simulink model "WSCC_9bus_distributed"  (R2018a)
settings: Solver=ode3  StartTime=0.0  StopTime=1  FixedStep=Ts  MaxStep=1e-4  RelTol=1e-3
InitFcn:
  | Ts=50e-6;
  | Freq=60;
undefined symbols (not defined in the file or in its folder): gcbh, i, phase, sps_rtmsupport
libraries: powerlib x105, spsVIMeasurementModel x81, library x28, sps_avr x9, CoSiF x7
(part 3 of 5)

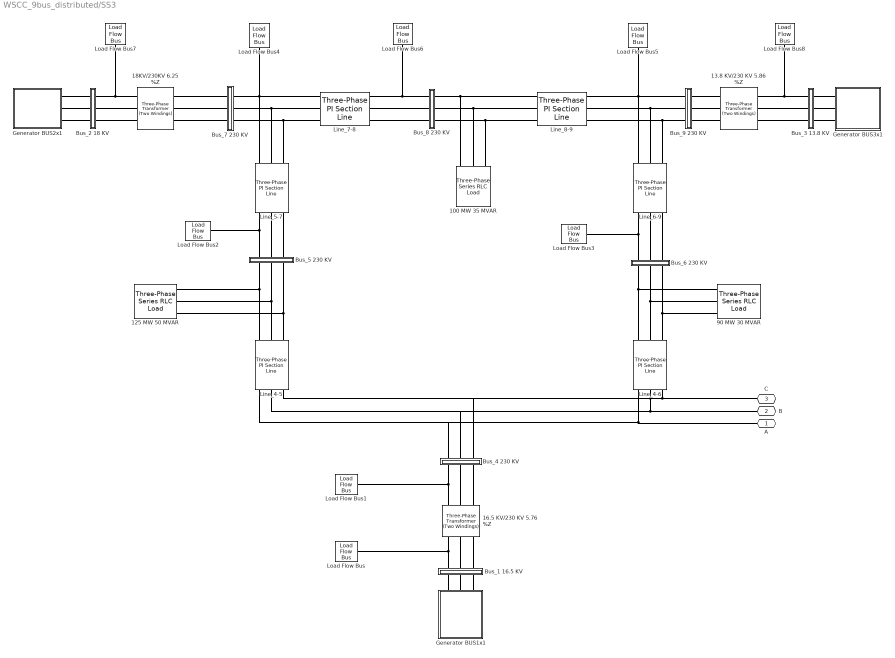
== system WSCC_9bus_distributed/SS3 ==
  100 MW 35 MVAR : powerlib/Elements/Three-Phase Series RLC Load  LConnTagsString=A|B|C  Configuration=Y (grounded)  NominalVoltage=(230000)*1.01601  Vabc=[1e3 1e3 1e3]  Vabcp=[1e3 1e3 1e3]  NominalFrequency=60  UnbalancedPower=off  ActivePower=100e6  InductivePower=35e6  CapacitivePower=0  Pabc=[10e3 9e3 11e3]  QLabc=[100 90 110]  QCabc=[100 90 110]  Pabcp=[10e3 9e3 11e3]  QLabcp=[100 90 110]  QCabcp=[100 90 110]  Measurements=Branch voltages and currents  LoadType=constant PQ
  125 MW 50 MVAR : powerlib/Elements/Three-Phase Series RLC Load  LConnTagsString=A|B|C  Configuration=Y (grounded)  NominalVoltage=(230000)*0.996126  Vabc=[1e3 1e3 1e3]  Vabcp=[1e3 1e3 1e3]  NominalFrequency=60  UnbalancedPower=off  ActivePower=125e6  InductivePower=50e6  CapacitivePower=0  Pabc=[10e3 9e3 11e3]  QLabc=[100 90 110]  QCabc=[100 90 110]  Pabcp=[10e3 9e3 11e3]  QLabcp=[100 90 110]  QCabcp=[100 90 110]  Measurements=Branch voltages and currents  LoadType=constant PQ
  13.8 KV/230 KV 5.86 %Z : powerlib/Elements/Three-Phase Transformer (Two Windings)  Winding1Connection=Yg  Winding2Connection=Yg  CoreType=Three single-phase transformers  SetSaturation=off  Hysteresis=off  DataFile='hysteresis'  SetInitialFlux=off  Measurements=None  UNITS=pu  NominalPower=[ 128e6 , 60 ]  Winding1=[ 13.8e3 , 1e-6 , 0.0 ]  Winding2=[ 230e3 , 1e-6, 0.075008 ]  Rm=inf  Lm=inf  L0=0.5  Saturation=[ 0,0 ; 0.0024,1.2 ; 1.0,1.52 ]  InitialFluxes=[ 0.8 , -0.8 , 0.7 ]  MoreParameters=off  BreakLoop=off  DataType=off  TransfoNumber=1
  "16.5 KV/230 KV 5.76 %Z     " : powerlib/Elements/Three-Phase Transformer (Two Windings)  Winding1Connection=Yg  Winding2Connection=Yg  CoreType=Three single-phase transformers  SetSaturation=off  Hysteresis=off  DataFile='hysteresis'  SetInitialFlux=off  Measurements=None  UNITS=pu  NominalPower=[ 247.5e6 , 60 ]  Winding1=[ 16.5e3 , 1e-6, 0.0 ]  Winding2=[ 230e3 ,1e-6, 0.14256 ]  Rm=inf  Lm=inf  L0=0.5  Saturation=[ 0,0 ; 0.0024,1.2 ; 1.0,1.52 ]  InitialFluxes=[ 0.8 , -0.8 , 0.7 ]  MoreParameters=off  BreakLoop=off  DataType=off  TransfoNumber=1
  18KV/230KV 6.25 %Z : powerlib/Elements/Three-Phase Transformer (Two Windings)  Winding1Connection=Yg  Winding2Connection=Yg  CoreType=Three single-phase transformers  SetSaturation=off  Hysteresis=off  DataFile='hysteresis'  SetInitialFlux=off  Measurements=None  UNITS=pu  NominalPower=[ 192e6 , 60 ]  Winding1=[ 18e3 , 1e-6 , 0.0 ]  Winding2=[ 230e3 , 1e-6, 0.12 ]  Rm=inf  Lm=inf  L0=0.5  Saturation=[ 0,0 ; 0.0024,1.2 ; 1.0,1.52 ]  InitialFluxes=[ 0.8 , -0.8 , 0.7 ]  MoreParameters=off  BreakLoop=off  DataType=off  TransfoNumber=1
  90 MW 30 MVAR : powerlib/Elements/Three-Phase Series RLC Load  LConnTagsString=A|B|C  Configuration=Y (grounded)  NominalVoltage=(230000)*1.01311  Vabc=[1e3 1e3 1e3]  Vabcp=[1e3 1e3 1e3]  NominalFrequency=60  UnbalancedPower=off  ActivePower=90e6  InductivePower=30e6  CapacitivePower=0  Pabc=[10e3 9e3 11e3]  QLabc=[100 90 110]  QCabc=[100 90 110]  Pabcp=[10e3 9e3 11e3]  QLabcp=[100 90 110]  QCabcp=[100 90 110]  Measurements=Branch voltages and currents  LoadType=constant PQ
  Bus_1 16.5 KV : Subsystem  DialogController=POWERSYS.PowerSysDialog  LoadFcn=sps_rtmsupport('LoadFcn',gcbh);  StartFcn=sps_rtmsupport('StartFcn',gcbh);  StopFcn=sps_rtmsupport('StopFcn',gcbh);  mask(Three-Phase VI Measurement){VoltageMeasurement=phase-to-phase, SetLabelV=on, LabelV=ss3_Vabc_1, Vpu=off, VpuLL=off, CurrentMeasurement=yes, SetLabelI=on, LabelI=ss3_Iabc_1, Ipu=off, Pbase=100e6, Vbase=16.5e3, OutputType=Complex, PhasorSimulation=off, PSBequivalent=0}
      mask prompts: VoltageMeasurement "Voltage measurement"; SetLabelV "Use a label"; LabelV "Signal label  (use a From block to collect this signal)"; Vpu "Voltages in pu,  based on peak value of nominal phase-to-ground voltage"; VpuLL "Voltages in pu,  based on peak value of nominal phase-to-phase  voltage"; CurrentMeasurement "Current measurement"; SetLabelI "Use a label"; LabelI "Signal label  (use a From block to collect this signal)"; Ipu "Currents in pu"; Pbase "Base power ( VA 3 phase)"; Vbase "Nominal voltage used for pu measurement (Vrms phase-phase) :"; OutputType "Output signals in:"; PhasorSimulation "Phasor simulation (internal use)"; PSBequivalent "Equivalent circuit (internal use)"
      mask help:
      | Ideal three-phase voltage and current measurements.
      |
      | The block can output the voltages and currents in per unit values or in volts and amperes.
      mask init: same as WSCC_9bus_distributed/SS1/Bus_1 16.5 KV
      settings: CopyFcn=sps_rtmsupport('CopyFcn',gcbh); powericon('ThreePhaseVIMeasurementCopy',gcb)  DeleteFcn=sps_rtmsupport('DeleteFcn',gcbh);  UndoDeleteFcn=sps_rtmsupport('UndoDeleteFcn',gcbh);  ModelCloseFcn=sps_rtmsupport('ModelCloseFcn',gcbh);  PreSaveFcn="sps_rtmsupport('PreSaveFcn',gcbh);  set_param(gcb,'LinkStatus','restore')"  PostSaveFcn=sps_rtmsupport('PostSaveFcn',gcbh);  NameChangeFcn=sps_rtmsupport('NameChangeFcn',gcbh);  PreCopyFcn=sps_rtmsupport('PreCopyFcn',gcbh);  OpenFcn=sps_rtmsupport('OpenFcn',gcbh, [1 2 4 5 6 7 9 -12 13]);  CloseFcn=sps_rtmsupport('CloseFcn',gcbh);  PreDeleteFcn=sps_rtmsupport('PreDeleteFcn',gcbh);
      mask Help: helpview(psbhelp)
      mask TypeOptions VoltageMeasurement: no | phase-to-ground | phase-to-phase
      mask Callback VoltageMeasurement: powericon('ThreePhaseVIMeasurementCback',gcb,'Vselector');
      mask Callback SetLabelV: powericon('ThreePhaseVIMeasurementCback',gcb,'');
      mask Callback Vpu: powericon('ThreePhaseVIMeasurementCback',gcb,'Vpu');
      mask Callback VpuLL: powericon('ThreePhaseVIMeasurementCback',gcb,'VpuLL');
      mask TypeOptions CurrentMeasurement: no | yes
      mask Callback CurrentMeasurement: powericon('ThreePhaseVIMeasurementCback',gcb,'');
      mask Callback SetLabelI: powericon('ThreePhaseVIMeasurementCback',gcb,'');
      mask Callback LabelI: powericon('ThreePhaseVIMeasurementCback',gcb,'');
      mask Callback Ipu: powericon('ThreePhaseVIMeasurementCback',gcb,'');
      mask TypeOptions OutputType: Complex | Real-Imag | Magnitude-Angle | Magnitude
  Bus_2 18 KV : Subsystem  DialogController=POWERSYS.PowerSysDialog  LoadFcn=sps_rtmsupport('LoadFcn',gcbh);  StartFcn=sps_rtmsupport('StartFcn',gcbh);  StopFcn=sps_rtmsupport('StopFcn',gcbh);  mask(Three-Phase VI Measurement){VoltageMeasurement=phase-to-phase, SetLabelV=on, LabelV=ss3_Vabc_2, Vpu=off, VpuLL=off, CurrentMeasurement=yes, SetLabelI=on, LabelI=ss3_Iabc_2, Ipu=off, Pbase=100e6, Vbase=18e3, OutputType=Complex, PhasorSimulation=off, PSBequivalent=0}
      mask prompts: VoltageMeasurement "Voltage measurement"; SetLabelV "Use a label"; LabelV "Signal label  (use a From block to collect this signal)"; Vpu "Voltages in pu,  based on peak value of nominal phase-to-ground voltage"; VpuLL "Voltages in pu,  based on peak value of nominal phase-to-phase  voltage"; CurrentMeasurement "Current measurement"; SetLabelI "Use a label"; LabelI "Signal label  (use a From block to collect this signal)"; Ipu "Currents in pu"; Pbase "Base power ( VA 3 phase)"; Vbase "Nominal voltage used for pu measurement (Vrms phase-phase) :"; OutputType "Output signals in:"; PhasorSimulation "Phasor simulation (internal use)"; PSBequivalent "Equivalent circuit (internal use)"
      mask help:
      | Ideal three-phase voltage and current measurements.
      |
      | The block can output the voltages and currents in per unit values or in volts and amperes.
      mask init: same as WSCC_9bus_distributed/SS1/Bus_1 16.5 KV
      settings: CopyFcn=sps_rtmsupport('CopyFcn',gcbh); powericon('ThreePhaseVIMeasurementCopy',gcb)  DeleteFcn=sps_rtmsupport('DeleteFcn',gcbh);  UndoDeleteFcn=sps_rtmsupport('UndoDeleteFcn',gcbh);  ModelCloseFcn=sps_rtmsupport('ModelCloseFcn',gcbh);  PreSaveFcn="sps_rtmsupport('PreSaveFcn',gcbh);  set_param(gcb,'LinkStatus','restore')"  PostSaveFcn=sps_rtmsupport('PostSaveFcn',gcbh);  NameChangeFcn=sps_rtmsupport('NameChangeFcn',gcbh);  PreCopyFcn=sps_rtmsupport('PreCopyFcn',gcbh);  OpenFcn=sps_rtmsupport('OpenFcn',gcbh, [1 2 4 5 6 7 9 -12 13]);  CloseFcn=sps_rtmsupport('CloseFcn',gcbh);  PreDeleteFcn=sps_rtmsupport('PreDeleteFcn',gcbh);
      mask Help: helpview(psbhelp)
      mask TypeOptions VoltageMeasurement: no | phase-to-ground | phase-to-phase
      mask Callback VoltageMeasurement: powericon('ThreePhaseVIMeasurementCback',gcb,'Vselector');
      mask Callback SetLabelV: powericon('ThreePhaseVIMeasurementCback',gcb,'');
      mask Callback Vpu: powericon('ThreePhaseVIMeasurementCback',gcb,'Vpu');
      mask Callback VpuLL: powericon('ThreePhaseVIMeasurementCback',gcb,'VpuLL');
      mask TypeOptions CurrentMeasurement: no | yes
      mask Callback CurrentMeasurement: powericon('ThreePhaseVIMeasurementCback',gcb,'');
      mask Callback SetLabelI: powericon('ThreePhaseVIMeasurementCback',gcb,'');
      mask Callback LabelI: powericon('ThreePhaseVIMeasurementCback',gcb,'');
      mask Callback Ipu: powericon('ThreePhaseVIMeasurementCback',gcb,'');
      mask TypeOptions OutputType: Complex | Real-Imag | Magnitude-Angle | Magnitude
  Bus_3 13.8 KV : Subsystem  DialogController=POWERSYS.PowerSysDialog  LoadFcn=sps_rtmsupport('LoadFcn',gcbh);  StartFcn=sps_rtmsupport('StartFcn',gcbh);  StopFcn=sps_rtmsupport('StopFcn',gcbh);  mask(Three-Phase VI Measurement){VoltageMeasurement=phase-to-phase, SetLabelV=on, LabelV=ss3_Vabc_3, Vpu=off, VpuLL=off, CurrentMeasurement=yes, SetLabelI=on, LabelI=ss3_Iabc_3, Ipu=off, Pbase=100e6, Vbase=13.8e3, OutputType=Complex, PhasorSimulation=off, PSBequivalent=0}
      mask prompts: VoltageMeasurement "Voltage measurement"; SetLabelV "Use a label"; LabelV "Signal label  (use a From block to collect this signal)"; Vpu "Voltages in pu,  based on peak value of nominal phase-to-ground voltage"; VpuLL "Voltages in pu,  based on peak value of nominal phase-to-phase  voltage"; CurrentMeasurement "Current measurement"; SetLabelI "Use a label"; LabelI "Signal label  (use a From block to collect this signal)"; Ipu "Currents in pu"; Pbase "Base power ( VA 3 phase)"; Vbase "Nominal voltage used for pu measurement (Vrms phase-phase) :"; OutputType "Output signals in:"; PhasorSimulation "Phasor simulation (internal use)"; PSBequivalent "Equivalent circuit (internal use)"
      mask help:
      | Ideal three-phase voltage and current measurements.
      |
      | The block can output the voltages and currents in per unit values or in volts and amperes.
      mask init: same as WSCC_9bus_distributed/SS1/Bus_1 16.5 KV
      settings: CopyFcn=sps_rtmsupport('CopyFcn',gcbh); powericon('ThreePhaseVIMeasurementCopy',gcb)  DeleteFcn=sps_rtmsupport('DeleteFcn',gcbh);  UndoDeleteFcn=sps_rtmsupport('UndoDeleteFcn',gcbh);  ModelCloseFcn=sps_rtmsupport('ModelCloseFcn',gcbh);  PreSaveFcn="sps_rtmsupport('PreSaveFcn',gcbh);  set_param(gcb,'LinkStatus','restore')"  PostSaveFcn=sps_rtmsupport('PostSaveFcn',gcbh);  NameChangeFcn=sps_rtmsupport('NameChangeFcn',gcbh);  PreCopyFcn=sps_rtmsupport('PreCopyFcn',gcbh);  OpenFcn=sps_rtmsupport('OpenFcn',gcbh, [1 2 4 5 6 7 9 -12 13]);  CloseFcn=sps_rtmsupport('CloseFcn',gcbh);  PreDeleteFcn=sps_rtmsupport('PreDeleteFcn',gcbh);
      mask Help: helpview(psbhelp)
      mask TypeOptions VoltageMeasurement: no | phase-to-ground | phase-to-phase
      mask Callback VoltageMeasurement: powericon('ThreePhaseVIMeasurementCback',gcb,'Vselector');
      mask Callback SetLabelV: powericon('ThreePhaseVIMeasurementCback',gcb,'');
      mask Callback Vpu: powericon('ThreePhaseVIMeasurementCback',gcb,'Vpu');
      mask Callback VpuLL: powericon('ThreePhaseVIMeasurementCback',gcb,'VpuLL');
      mask TypeOptions CurrentMeasurement: no | yes
      mask Callback CurrentMeasurement: powericon('ThreePhaseVIMeasurementCback',gcb,'');
      mask Callback SetLabelI: powericon('ThreePhaseVIMeasurementCback',gcb,'');
      mask Callback LabelI: powericon('ThreePhaseVIMeasurementCback',gcb,'');
      mask Callback Ipu: powericon('ThreePhaseVIMeasurementCback',gcb,'');
      mask TypeOptions OutputType: Complex | Real-Imag | Magnitude-Angle | Magnitude
  Bus_4 230 KV : Subsystem  DialogController=POWERSYS.PowerSysDialog  LoadFcn=sps_rtmsupport('LoadFcn',gcbh);  StartFcn=sps_rtmsupport('StartFcn',gcbh);  StopFcn=sps_rtmsupport('StopFcn',gcbh);  mask(Three-Phase VI Measurement){VoltageMeasurement=phase-to-phase, SetLabelV=on, LabelV=ss3_Vabc_4, Vpu=off, VpuLL=off, CurrentMeasurement=yes, SetLabelI=on, LabelI=ss3_Iabc_4, Ipu=off, Pbase=100e6, Vbase=230e3, OutputType=Complex, PhasorSimulation=off, PSBequivalent=0}
      mask prompts: VoltageMeasurement "Voltage measurement"; SetLabelV "Use a label"; LabelV "Signal label  (use a From block to collect this signal)"; Vpu "Voltages in pu,  based on peak value of nominal phase-to-ground voltage"; VpuLL "Voltages in pu,  based on peak value of nominal phase-to-phase  voltage"; CurrentMeasurement "Current measurement"; SetLabelI "Use a label"; LabelI "Signal label  (use a From block to collect this signal)"; Ipu "Currents in pu"; Pbase "Base power ( VA 3 phase)"; Vbase "Nominal voltage used for pu measurement (Vrms phase-phase) :"; OutputType "Output signals in:"; PhasorSimulation "Phasor simulation (internal use)"; PSBequivalent "Equivalent circuit (internal use)"
      mask help:
      | Ideal three-phase voltage and current measurements.
      |
      | The block can output the voltages and currents in per unit values or in volts and amperes.
      mask init: same as WSCC_9bus_distributed/SS1/Bus_1 16.5 KV
      settings: CopyFcn=sps_rtmsupport('CopyFcn',gcbh); powericon('ThreePhaseVIMeasurementCopy',gcb)  DeleteFcn=sps_rtmsupport('DeleteFcn',gcbh);  UndoDeleteFcn=sps_rtmsupport('UndoDeleteFcn',gcbh);  ModelCloseFcn=sps_rtmsupport('ModelCloseFcn',gcbh);  PreSaveFcn="sps_rtmsupport('PreSaveFcn',gcbh);  set_param(gcb,'LinkStatus','restore')"  PostSaveFcn=sps_rtmsupport('PostSaveFcn',gcbh);  NameChangeFcn=sps_rtmsupport('NameChangeFcn',gcbh);  PreCopyFcn=sps_rtmsupport('PreCopyFcn',gcbh);  OpenFcn=sps_rtmsupport('OpenFcn',gcbh, [1 2 4 5 6 7 9 -12 13]);  CloseFcn=sps_rtmsupport('CloseFcn',gcbh);  PreDeleteFcn=sps_rtmsupport('PreDeleteFcn',gcbh);
      mask Help: helpview(psbhelp)
      mask TypeOptions VoltageMeasurement: no | phase-to-ground | phase-to-phase
      mask Callback VoltageMeasurement: powericon('ThreePhaseVIMeasurementCback',gcb,'Vselector');
      mask Callback SetLabelV: powericon('ThreePhaseVIMeasurementCback',gcb,'');
      mask Callback Vpu: powericon('ThreePhaseVIMeasurementCback',gcb,'Vpu');
      mask Callback VpuLL: powericon('ThreePhaseVIMeasurementCback',gcb,'VpuLL');
      mask TypeOptions CurrentMeasurement: no | yes
      mask Callback CurrentMeasurement: powericon('ThreePhaseVIMeasurementCback',gcb,'');
      mask Callback SetLabelI: powericon('ThreePhaseVIMeasurementCback',gcb,'');
      mask Callback LabelI: powericon('ThreePhaseVIMeasurementCback',gcb,'');
      mask Callback Ipu: powericon('ThreePhaseVIMeasurementCback',gcb,'');
      mask TypeOptions OutputType: Complex | Real-Imag | Magnitude-Angle | Magnitude
  Bus_5 230 KV : Subsystem  DialogController=POWERSYS.PowerSysDialog  LoadFcn=sps_rtmsupport('LoadFcn',gcbh);  StartFcn=sps_rtmsupport('StartFcn',gcbh);  StopFcn=sps_rtmsupport('StopFcn',gcbh);  mask(Three-Phase VI Measurement){VoltageMeasurement=phase-to-phase, SetLabelV=on, LabelV=ss3_Vabc_5, Vpu=off, VpuLL=off, CurrentMeasurement=yes, SetLabelI=on, LabelI=ss3_Iabc_5, Ipu=off, Pbase=100e6, Vbase=230e3, OutputType=Complex, PhasorSimulation=off, PSBequivalent=0}
      mask prompts: VoltageMeasurement "Voltage measurement"; SetLabelV "Use a label"; LabelV "Signal label  (use a From block to collect this signal)"; Vpu "Voltages in pu,  based on peak value of nominal phase-to-ground voltage"; VpuLL "Voltages in pu,  based on peak value of nominal phase-to-phase  voltage"; CurrentMeasurement "Current measurement"; SetLabelI "Use a label"; LabelI "Signal label  (use a From block to collect this signal)"; Ipu "Currents in pu"; Pbase "Base power ( VA 3 phase)"; Vbase "Nominal voltage used for pu measurement (Vrms phase-phase) :"; OutputType "Output signals in:"; PhasorSimulation "Phasor simulation (internal use)"; PSBequivalent "Equivalent circuit (internal use)"
      mask help:
      | Ideal three-phase voltage and current measurements.
      |
      | The block can output the voltages and currents in per unit values or in volts and amperes.
      mask init: same as WSCC_9bus_distributed/SS1/Bus_1 16.5 KV
      settings: CopyFcn=sps_rtmsupport('CopyFcn',gcbh); powericon('ThreePhaseVIMeasurementCopy',gcb)  DeleteFcn=sps_rtmsupport('DeleteFcn',gcbh);  UndoDeleteFcn=sps_rtmsupport('UndoDeleteFcn',gcbh);  ModelCloseFcn=sps_rtmsupport('ModelCloseFcn',gcbh);  PreSaveFcn="sps_rtmsupport('PreSaveFcn',gcbh);  set_param(gcb,'LinkStatus','restore')"  PostSaveFcn=sps_rtmsupport('PostSaveFcn',gcbh);  NameChangeFcn=sps_rtmsupport('NameChangeFcn',gcbh);  PreCopyFcn=sps_rtmsupport('PreCopyFcn',gcbh);  OpenFcn=sps_rtmsupport('OpenFcn',gcbh, [1 2 4 5 6 7 9 -12 13]);  CloseFcn=sps_rtmsupport('CloseFcn',gcbh);  PreDeleteFcn=sps_rtmsupport('PreDeleteFcn',gcbh);
      mask Help: helpview(psbhelp)
      mask TypeOptions VoltageMeasurement: no | phase-to-ground | phase-to-phase
      mask Callback VoltageMeasurement: powericon('ThreePhaseVIMeasurementCback',gcb,'Vselector');
      mask Callback SetLabelV: powericon('ThreePhaseVIMeasurementCback',gcb,'');
      mask Callback Vpu: powericon('ThreePhaseVIMeasurementCback',gcb,'Vpu');
      mask Callback VpuLL: powericon('ThreePhaseVIMeasurementCback',gcb,'VpuLL');
      mask TypeOptions CurrentMeasurement: no | yes
      mask Callback CurrentMeasurement: powericon('ThreePhaseVIMeasurementCback',gcb,'');
      mask Callback SetLabelI: powericon('ThreePhaseVIMeasurementCback',gcb,'');
      mask Callback LabelI: powericon('ThreePhaseVIMeasurementCback',gcb,'');
      mask Callback Ipu: powericon('ThreePhaseVIMeasurementCback',gcb,'');
      mask TypeOptions OutputType: Complex | Real-Imag | Magnitude-Angle | Magnitude
  Bus_6 230 KV : Subsystem  DialogController=POWERSYS.PowerSysDialog  LoadFcn=sps_rtmsupport('LoadFcn',gcbh);  StartFcn=sps_rtmsupport('StartFcn',gcbh);  StopFcn=sps_rtmsupport('StopFcn',gcbh);  mask(Three-Phase VI Measurement){VoltageMeasurement=phase-to-phase, SetLabelV=on, LabelV=ss3_Vabc_6, Vpu=off, VpuLL=off, CurrentMeasurement=yes, SetLabelI=on, LabelI=ss3_Iabc_6, Ipu=off, Pbase=100e6, Vbase=230e3, OutputType=Complex, PhasorSimulation=off, PSBequivalent=0}
      mask prompts: VoltageMeasurement "Voltage measurement"; SetLabelV "Use a label"; LabelV "Signal label  (use a From block to collect this signal)"; Vpu "Voltages in pu,  based on peak value of nominal phase-to-ground voltage"; VpuLL "Voltages in pu,  based on peak value of nominal phase-to-phase  voltage"; CurrentMeasurement "Current measurement"; SetLabelI "Use a label"; LabelI "Signal label  (use a From block to collect this signal)"; Ipu "Currents in pu"; Pbase "Base power ( VA 3 phase)"; Vbase "Nominal voltage used for pu measurement (Vrms phase-phase) :"; OutputType "Output signals in:"; PhasorSimulation "Phasor simulation (internal use)"; PSBequivalent "Equivalent circuit (internal use)"
      mask help:
      | Ideal three-phase voltage and current measurements.
      |
      | The block can output the voltages and currents in per unit values or in volts and amperes.
      mask init: same as WSCC_9bus_distributed/SS1/Bus_1 16.5 KV
      settings: CopyFcn=sps_rtmsupport('CopyFcn',gcbh); powericon('ThreePhaseVIMeasurementCopy',gcb)  DeleteFcn=sps_rtmsupport('DeleteFcn',gcbh);  UndoDeleteFcn=sps_rtmsupport('UndoDeleteFcn',gcbh);  ModelCloseFcn=sps_rtmsupport('ModelCloseFcn',gcbh);  PreSaveFcn="sps_rtmsupport('PreSaveFcn',gcbh);  set_param(gcb,'LinkStatus','restore')"  PostSaveFcn=sps_rtmsupport('PostSaveFcn',gcbh);  NameChangeFcn=sps_rtmsupport('NameChangeFcn',gcbh);  PreCopyFcn=sps_rtmsupport('PreCopyFcn',gcbh);  OpenFcn=sps_rtmsupport('OpenFcn',gcbh, [1 2 4 5 6 7 9 -12 13]);  CloseFcn=sps_rtmsupport('CloseFcn',gcbh);  PreDeleteFcn=sps_rtmsupport('PreDeleteFcn',gcbh);
      mask Help: helpview(psbhelp)
      mask TypeOptions VoltageMeasurement: no | phase-to-ground | phase-to-phase
      mask Callback VoltageMeasurement: powericon('ThreePhaseVIMeasurementCback',gcb,'Vselector');
      mask Callback SetLabelV: powericon('ThreePhaseVIMeasurementCback',gcb,'');
      mask Callback Vpu: powericon('ThreePhaseVIMeasurementCback',gcb,'Vpu');
      mask Callback VpuLL: powericon('ThreePhaseVIMeasurementCback',gcb,'VpuLL');
      mask TypeOptions CurrentMeasurement: no | yes
      mask Callback CurrentMeasurement: powericon('ThreePhaseVIMeasurementCback',gcb,'');
      mask Callback SetLabelI: powericon('ThreePhaseVIMeasurementCback',gcb,'');
      mask Callback LabelI: powericon('ThreePhaseVIMeasurementCback',gcb,'');
      mask Callback Ipu: powericon('ThreePhaseVIMeasurementCback',gcb,'');
      mask TypeOptions OutputType: Complex | Real-Imag | Magnitude-Angle | Magnitude
  "Bus_7 230 KV " : Subsystem  DialogController=POWERSYS.PowerSysDialog  LoadFcn=sps_rtmsupport('LoadFcn',gcbh);  StartFcn=sps_rtmsupport('StartFcn',gcbh);  StopFcn=sps_rtmsupport('StopFcn',gcbh);  mask(Three-Phase VI Measurement){VoltageMeasurement=phase-to-phase, SetLabelV=on, LabelV=ss3_Vabc_7, Vpu=off, VpuLL=off, CurrentMeasurement=yes, SetLabelI=on, LabelI=ss3_Iabc_7, Ipu=off, Pbase=100e6, Vbase=230e3, OutputType=Complex, PhasorSimulation=off, PSBequivalent=0}
      mask prompts: VoltageMeasurement "Voltage measurement"; SetLabelV "Use a label"; LabelV "Signal label  (use a From block to collect this signal)"; Vpu "Voltages in pu,  based on peak value of nominal phase-to-ground voltage"; VpuLL "Voltages in pu,  based on peak value of nominal phase-to-phase  voltage"; CurrentMeasurement "Current measurement"; SetLabelI "Use a label"; LabelI "Signal label  (use a From block to collect this signal)"; Ipu "Currents in pu"; Pbase "Base power ( VA 3 phase)"; Vbase "Nominal voltage used for pu measurement (Vrms phase-phase) :"; OutputType "Output signals in:"; PhasorSimulation "Phasor simulation (internal use)"; PSBequivalent "Equivalent circuit (internal use)"
      mask help:
      | Ideal three-phase voltage and current measurements.
      |
      | The block can output the voltages and currents in per unit values or in volts and amperes.
      mask init: same as WSCC_9bus_distributed/SS1/Bus_1 16.5 KV
      settings: CopyFcn=sps_rtmsupport('CopyFcn',gcbh); powericon('ThreePhaseVIMeasurementCopy',gcb)  DeleteFcn=sps_rtmsupport('DeleteFcn',gcbh);  UndoDeleteFcn=sps_rtmsupport('UndoDeleteFcn',gcbh);  ModelCloseFcn=sps_rtmsupport('ModelCloseFcn',gcbh);  PreSaveFcn="sps_rtmsupport('PreSaveFcn',gcbh);  set_param(gcb,'LinkStatus','restore')"  PostSaveFcn=sps_rtmsupport('PostSaveFcn',gcbh);  NameChangeFcn=sps_rtmsupport('NameChangeFcn',gcbh);  PreCopyFcn=sps_rtmsupport('PreCopyFcn',gcbh);  OpenFcn=sps_rtmsupport('OpenFcn',gcbh, [1 2 4 5 6 7 9 -12 13]);  CloseFcn=sps_rtmsupport('CloseFcn',gcbh);  PreDeleteFcn=sps_rtmsupport('PreDeleteFcn',gcbh);
      mask Help: helpview(psbhelp)
      mask TypeOptions VoltageMeasurement: no | phase-to-ground | phase-to-phase
      mask Callback VoltageMeasurement: powericon('ThreePhaseVIMeasurementCback',gcb,'Vselector');
      mask Callback SetLabelV: powericon('ThreePhaseVIMeasurementCback',gcb,'');
      mask Callback Vpu: powericon('ThreePhaseVIMeasurementCback',gcb,'Vpu');
      mask Callback VpuLL: powericon('ThreePhaseVIMeasurementCback',gcb,'VpuLL');
      mask TypeOptions CurrentMeasurement: no | yes
      mask Callback CurrentMeasurement: powericon('ThreePhaseVIMeasurementCback',gcb,'');
      mask Callback SetLabelI: powericon('ThreePhaseVIMeasurementCback',gcb,'');
      mask Callback LabelI: powericon('ThreePhaseVIMeasurementCback',gcb,'');
      mask Callback Ipu: powericon('ThreePhaseVIMeasurementCback',gcb,'');
      mask TypeOptions OutputType: Complex | Real-Imag | Magnitude-Angle | Magnitude
  Bus_8 230 KV : Subsystem  DialogController=POWERSYS.PowerSysDialog  LoadFcn=sps_rtmsupport('LoadFcn',gcbh);  StartFcn=sps_rtmsupport('StartFcn',gcbh);  StopFcn=sps_rtmsupport('StopFcn',gcbh);  mask(Three-Phase VI Measurement){VoltageMeasurement=phase-to-phase, SetLabelV=on, LabelV=ss3_Vabc_8, Vpu=off, VpuLL=off, CurrentMeasurement=yes, SetLabelI=on, LabelI=ss3_Iabc_8, Ipu=off, Pbase=100e6, Vbase=230e3, OutputType=Complex, PhasorSimulation=off, PSBequivalent=0}
      mask prompts: VoltageMeasurement "Voltage measurement"; SetLabelV "Use a label"; LabelV "Signal label  (use a From block to collect this signal)"; Vpu "Voltages in pu,  based on peak value of nominal phase-to-ground voltage"; VpuLL "Voltages in pu,  based on peak value of nominal phase-to-phase  voltage"; CurrentMeasurement "Current measurement"; SetLabelI "Use a label"; LabelI "Signal label  (use a From block to collect this signal)"; Ipu "Currents in pu"; Pbase "Base power ( VA 3 phase)"; Vbase "Nominal voltage used for pu measurement (Vrms phase-phase) :"; OutputType "Output signals in:"; PhasorSimulation "Phasor simulation (internal use)"; PSBequivalent "Equivalent circuit (internal use)"
      mask help:
      | Ideal three-phase voltage and current measurements.
      |
      | The block can output the voltages and currents in per unit values or in volts and amperes.
      mask init: same as WSCC_9bus_distributed/SS1/Bus_1 16.5 KV
      settings: CopyFcn=sps_rtmsupport('CopyFcn',gcbh); powericon('ThreePhaseVIMeasurementCopy',gcb)  DeleteFcn=sps_rtmsupport('DeleteFcn',gcbh);  UndoDeleteFcn=sps_rtmsupport('UndoDeleteFcn',gcbh);  ModelCloseFcn=sps_rtmsupport('ModelCloseFcn',gcbh);  PreSaveFcn="sps_rtmsupport('PreSaveFcn',gcbh);  set_param(gcb,'LinkStatus','restore')"  PostSaveFcn=sps_rtmsupport('PostSaveFcn',gcbh);  NameChangeFcn=sps_rtmsupport('NameChangeFcn',gcbh);  PreCopyFcn=sps_rtmsupport('PreCopyFcn',gcbh);  OpenFcn=sps_rtmsupport('OpenFcn',gcbh, [1 2 4 5 6 7 9 -12 13]);  CloseFcn=sps_rtmsupport('CloseFcn',gcbh);  PreDeleteFcn=sps_rtmsupport('PreDeleteFcn',gcbh);
      mask Help: helpview(psbhelp)
      mask TypeOptions VoltageMeasurement: no | phase-to-ground | phase-to-phase
      mask Callback VoltageMeasurement: powericon('ThreePhaseVIMeasurementCback',gcb,'Vselector');
      mask Callback SetLabelV: powericon('ThreePhaseVIMeasurementCback',gcb,'');
      mask Callback Vpu: powericon('ThreePhaseVIMeasurementCback',gcb,'Vpu');
      mask Callback VpuLL: powericon('ThreePhaseVIMeasurementCback',gcb,'VpuLL');
      mask TypeOptions CurrentMeasurement: no | yes
      mask Callback CurrentMeasurement: powericon('ThreePhaseVIMeasurementCback',gcb,'');
      mask Callback SetLabelI: powericon('ThreePhaseVIMeasurementCback',gcb,'');
      mask Callback LabelI: powericon('ThreePhaseVIMeasurementCback',gcb,'');
      mask Callback Ipu: powericon('ThreePhaseVIMeasurementCback',gcb,'');
      mask TypeOptions OutputType: Complex | Real-Imag | Magnitude-Angle | Magnitude
  Bus_9 230 KV : Subsystem  DialogController=POWERSYS.PowerSysDialog  LoadFcn=sps_rtmsupport('LoadFcn',gcbh);  StartFcn=sps_rtmsupport('StartFcn',gcbh);  StopFcn=sps_rtmsupport('StopFcn',gcbh);  mask(Three-Phase VI Measurement){VoltageMeasurement=phase-to-phase, SetLabelV=on, LabelV=ss3_Vabc_9, Vpu=off, VpuLL=off, CurrentMeasurement=yes, SetLabelI=on, LabelI=ss3_Iabc_9, Ipu=off, Pbase=100e6, Vbase=230e3, OutputType=Complex, PhasorSimulation=off, PSBequivalent=0}
      mask prompts: VoltageMeasurement "Voltage measurement"; SetLabelV "Use a label"; LabelV "Signal label  (use a From block to collect this signal)"; Vpu "Voltages in pu,  based on peak value of nominal phase-to-ground voltage"; VpuLL "Voltages in pu,  based on peak value of nominal phase-to-phase  voltage"; CurrentMeasurement "Current measurement"; SetLabelI "Use a label"; LabelI "Signal label  (use a From block to collect this signal)"; Ipu "Currents in pu"; Pbase "Base power ( VA 3 phase)"; Vbase "Nominal voltage used for pu measurement (Vrms phase-phase) :"; OutputType "Output signals in:"; PhasorSimulation "Phasor simulation (internal use)"; PSBequivalent "Equivalent circuit (internal use)"
      mask help:
      | Ideal three-phase voltage and current measurements.
      |
      | The block can output the voltages and currents in per unit values or in volts and amperes.
      mask init: same as WSCC_9bus_distributed/SS1/Bus_1 16.5 KV
      settings: CopyFcn=sps_rtmsupport('CopyFcn',gcbh); powericon('ThreePhaseVIMeasurementCopy',gcb)  DeleteFcn=sps_rtmsupport('DeleteFcn',gcbh);  UndoDeleteFcn=sps_rtmsupport('UndoDeleteFcn',gcbh);  ModelCloseFcn=sps_rtmsupport('ModelCloseFcn',gcbh);  PreSaveFcn="sps_rtmsupport('PreSaveFcn',gcbh);  set_param(gcb,'LinkStatus','restore')"  PostSaveFcn=sps_rtmsupport('PostSaveFcn',gcbh);  NameChangeFcn=sps_rtmsupport('NameChangeFcn',gcbh);  PreCopyFcn=sps_rtmsupport('PreCopyFcn',gcbh);  OpenFcn=sps_rtmsupport('OpenFcn',gcbh, [1 2 4 5 6 7 9 -12 13]);  CloseFcn=sps_rtmsupport('CloseFcn',gcbh);  PreDeleteFcn=sps_rtmsupport('PreDeleteFcn',gcbh);
      mask Help: helpview(psbhelp)
      mask TypeOptions VoltageMeasurement: no | phase-to-ground | phase-to-phase
      mask Callback VoltageMeasurement: powericon('ThreePhaseVIMeasurementCback',gcb,'Vselector');
      mask Callback SetLabelV: powericon('ThreePhaseVIMeasurementCback',gcb,'');
      mask Callback Vpu: powericon('ThreePhaseVIMeasurementCback',gcb,'Vpu');
      mask Callback VpuLL: powericon('ThreePhaseVIMeasurementCback',gcb,'VpuLL');
      mask TypeOptions CurrentMeasurement: no | yes
      mask Callback CurrentMeasurement: powericon('ThreePhaseVIMeasurementCback',gcb,'');
      mask Callback SetLabelI: powericon('ThreePhaseVIMeasurementCback',gcb,'');
      mask Callback LabelI: powericon('ThreePhaseVIMeasurementCback',gcb,'');
      mask Callback Ipu: powericon('ThreePhaseVIMeasurementCback',gcb,'');
      mask TypeOptions OutputType: Complex | Real-Imag | Magnitude-Angle | Magnitude
  Generator BUS1x1 : Subsystem
  Generator BUS2x1 : Subsystem
  Generator BUS3x1 : Subsystem
  Line_4-5 : powerlib/Elements/Three-Phase PI Section Line  LConnTagsString=a|b|c  RConnTagsString=A|B|C  Frequency=60  Resistances=[ 0.0529 0.13225]  Inductances="[ 1.192e-3  2.38e-3]"  Capacitances=[8.82e-9 5.188e-9]  Length=100
      settings: SourceProductName=Simscape Power Systems
  Line_4-6 : powerlib/Elements/Three-Phase PI Section Line  LConnTagsString=a|b|c  RConnTagsString=A|B|C  Frequency=60  Resistances=[ 0.08993 0.224825]  Inductances="[ 1.29e-3  3.22e-3]"  Capacitances=[7.922e-9 4.74e-9]  Length=100
      settings: SourceProductName=Simscape Power Systems
  Line_5-7 : powerlib/Elements/Three-Phase PI Section Line  LConnTagsString=a|b|c  RConnTagsString=A|B|C  Frequency=60  Resistances=[ 0.16928 0.4232]  Inductances="[ 2.259e-3  5.64e-3]"  Capacitances=[15.34e-9 9.025e-9]  Length=100
      settings: SourceProductName=Simscape Power Systems
  Line_6-9 : powerlib/Elements/Three-Phase PI Section Line  LConnTagsString=a|b|c  RConnTagsString=A|B|C  Frequency=60  Resistances=[ 0.20631 0.5157]  Inductances="[ 2.38e-3  6.09e-3]"  Capacitances=[17.95e-9 10.55e-9]  Length=100
      settings: SourceProductName=Simscape Power Systems
  Line_7-8 : powerlib/Elements/Three-Phase PI Section Line  LConnTagsString=a|b|c  RConnTagsString=A|B|C  Frequency=60  Resistances=[0.044965 0.11241]  Inductances="[ 1.01e-3  2.02e-3]"  Capacitances=[7.471e-9 4.394e-9]  Length=100
      settings: SourceProductName=Simscape Power Systems
  Line_8-9 : powerlib/Elements/Three-Phase PI Section Line  LConnTagsString=a|b|c  RConnTagsString=A|B|C  Frequency=60  Resistances=[ 0.062951 0.15737]  Inductances="[ 1.414e-3  3.53e-3]"  Capacitances=[10.47e-9 6.15e-9]  Length=100
      settings: SourceProductName=Simscape Power Systems
  Load Flow Bus : powerlib/Measurements/Load Flow Bus  LConnTagsString=a  Phases=single  Connectors=on one side  ID=ss3_BUS_1  Vbase=16.5e3  Vref=1.04  Vangle=0  VLF=1.04  VLFb=1  VLFc=1  angleLF=0  angleLFb=0  angleLFc=0
      settings: AttributesFormatString=%<ID>\n%<Vbase>V\n%<VLF>pu\n%<angleLF>deg.  SourceProductName=Simscape Power Systems
  Load Flow Bus1 : powerlib/Measurements/Load Flow Bus  LConnTagsString=a  Phases=single  Connectors=on one side  ID=ss3_BUS_4  Vbase=230e3  Vref=1  Vangle=0  VLF=1.026  VLFb=1  VLFc=1  angleLF=-2.214  angleLFb=0  angleLFc=0
      settings: AttributesFormatString=%<ID>\n%<Vbase>V\n%<VLF>pu\n%<angleLF>deg.  SourceProductName=Simscape Power Systems
  Load Flow Bus2 : powerlib/Measurements/Load Flow Bus  LConnTagsString=a  Phases=single  Connectors=on one side  ID=ss3_BUS_5  Vbase=230e3  Vref=1  Vangle=0  VLF=0.9961  VLFb=1  VLFc=1  angleLF=-3.98  angleLFb=0  angleLFc=0
      settings: AttributesFormatString=%<ID>\n%<Vbase>V\n%<VLF>pu\n%<angleLF>deg.  SourceProductName=Simscape Power Systems
  Load Flow Bus3 : powerlib/Measurements/Load Flow Bus  LConnTagsString=a  Phases=single  Connectors=on one side  ID=ss3_BUS_6  Vbase=230e3  Vref=1  Vangle=0  VLF=1.013  VLFb=1  VLFc=1  angleLF=-3.678  angleLFb=0  angleLFc=0
      settings: AttributesFormatString=%<ID>\n%<Vbase>V\n%<VLF>pu\n%<angleLF>deg.  SourceProductName=Simscape Power Systems
  Load Flow Bus4 : powerlib/Measurements/Load Flow Bus  LConnTagsString=a  Phases=single  Connectors=on one side  ID=ss3_BUS_7  Vbase=230e3  Vref=1  Vangle=0  VLF=1.026  VLFb=1  VLFc=1  angleLF=3.662  angleLFb=0  angleLFc=0
      settings: AttributesFormatString=%<ID>\n%<Vbase>V\n%<VLF>pu\n%<angleLF>deg.  SourceProductName=Simscape Power Systems
  Load Flow Bus5 : powerlib/Measurements/Load Flow Bus  LConnTagsString=a  Phases=single  Connectors=on one side  ID=ss3_BUS_9  Vbase=230e3  Vref=1  Vangle=0  VLF=1.032  VLFb=1  VLFc=1  angleLF=1.909  angleLFb=0  angleLFc=0
      settings: AttributesFormatString=%<ID>\n%<Vbase>V\n%<VLF>pu\n%<angleLF>deg.  SourceProductName=Simscape Power Systems
  Load Flow Bus6 : powerlib/Measurements/Load Flow Bus  LConnTagsString=a  Phases=single  Connectors=on one side  ID=ss3_BUS_8  Vbase=230e3  Vref=1  Vangle=0  VLF=1.016  VLFb=1  VLFc=1  angleLF=0.6755  angleLFb=0  angleLFc=0
      settings: AttributesFormatString=%<ID>\n%<Vbase>V\n%<VLF>pu\n%<angleLF>deg.  SourceProductName=Simscape Power Systems
  Load Flow Bus7 : powerlib/Measurements/Load Flow Bus  LConnTagsString=a  Phases=single  Connectors=on one side  ID=ss3_BUS_2  Vbase=18e3  Vref=1.025  Vangle=0  VLF=1.025  VLFb=1  VLFc=1  angleLF=9.222  angleLFb=0  angleLFc=0
      settings: AttributesFormatString=%<ID>\n%<Vbase>V\n%<VLF>pu\n%<angleLF>deg.  SourceProductName=Simscape Power Systems
  Load Flow Bus8 : powerlib/Measurements/Load Flow Bus  LConnTagsString=a  Phases=single  Connectors=on one side  ID=ss3_BUS_3  Vbase=13.8e3  Vref=1.025  Vangle=4.7  VLF=1.025  VLFb=1  VLFc=1  angleLF=4.606  angleLFb=0  angleLFc=0
      settings: AttributesFormatString=%<ID>\n%<Vbase>V\n%<VLF>pu\n%<angleLF>deg.  SourceProductName=Simscape Power Systems
  A : PMIOPort  Side=Left
  B : PMIOPort  Port=2  Side=Left
  C : PMIOPort  Port=3  Side=Left
  connections:
  Generator BUS3x1/RConn2 -- Bus_3 13.8 KV/RConn2
  Bus_4 230 KV/LConn2 -- "16.5 KV/230 KV 5.76 %Z     "/RConn2
  Line_6-9/RConn2 -- Bus_9 230 KV/LConn2 -- Line_8-9/RConn2
  Generator BUS1x1/RConn3 -- Bus_1 16.5 KV/RConn3
  Line_8-9/RConn1 -- Line_6-9/RConn1 -- Load Flow Bus5/LConn1 -- Bus_9 230 KV/LConn1
  Line_4-6/RConn3 -- 90 MW 30 MVAR/LConn3 -- Bus_6 230 KV/RConn3
  Bus_9 230 KV/RConn1 -- 13.8 KV/230 KV 5.86 %Z/RConn1
  Line_4-6/LConn2 -- Line_4-5/LConn2 -- Bus_4 230 KV/RConn2 -- B/RConn1
  "16.5 KV/230 KV 5.76 %Z     "/RConn3 -- Bus_4 230 KV/LConn3
  Line_6-9/RConn3 -- Line_8-9/RConn3 -- Bus_9 230 KV/LConn3
  Load Flow Bus1/LConn1 -- "16.5 KV/230 KV 5.76 %Z     "/RConn1 -- Bus_4 230 KV/LConn1
  Generator BUS2x1/RConn3 -- Bus_2 18 KV/LConn3
  18KV/230KV 6.25 %Z/RConn1 -- "Bus_7 230 KV "/LConn1
  18KV/230KV 6.25 %Z/RConn2 -- "Bus_7 230 KV "/LConn2
  18KV/230KV 6.25 %Z/RConn3 -- "Bus_7 230 KV "/LConn3
  Line_5-7/LConn1 -- Load Flow Bus2/LConn1 -- Bus_5 230 KV/LConn1
  Bus_6 230 KV/LConn1 -- Line_6-9/LConn1 -- Load Flow Bus3/LConn1
  Generator BUS3x1/RConn3 -- Bus_3 13.8 KV/RConn3
  Bus_9 230 KV/RConn3 -- 13.8 KV/230 KV 5.86 %Z/RConn3
  Generator BUS2x1/RConn2 -- Bus_2 18 KV/LConn2
  13.8 KV/230 KV 5.86 %Z/LConn3 -- Bus_3 13.8 KV/LConn3
  Line_7-8/RConn2 -- Bus_8 230 KV/RConn2
  Generator BUS2x1/RConn1 -- Bus_2 18 KV/LConn1
  Generator BUS1x1/RConn2 -- Bus_1 16.5 KV/RConn2
  A/RConn1 -- Line_4-5/LConn1 -- Bus_4 230 KV/RConn1 -- Line_4-6/LConn1
  Line_6-9/LConn3 -- Bus_6 230 KV/LConn3
  Line_4-6/RConn2 -- 90 MW 30 MVAR/LConn2 -- Bus_6 230 KV/RConn2
  18KV/230KV 6.25 %Z/LConn2 -- Bus_2 18 KV/RConn2
  Load Flow Bus7/LConn1 -- Bus_2 18 KV/RConn1 -- 18KV/230KV 6.25 %Z/LConn1
  100 MW 35 MVAR/LConn3 -- Line_8-9/LConn3 -- Bus_8 230 KV/LConn3
  Load Flow Bus8/LConn1 -- 13.8 KV/230 KV 5.86 %Z/LConn1 -- Bus_3 13.8 KV/LConn1
  100 MW 35 MVAR/LConn1 -- Line_8-9/LConn1 -- Bus_8 230 KV/LConn1
  Bus_8 230 KV/RConn1 -- Load Flow Bus6/LConn1 -- Line_7-8/RConn1
  Line_5-7/LConn3 -- Bus_5 230 KV/LConn3
  13.8 KV/230 KV 5.86 %Z/LConn2 -- Bus_3 13.8 KV/LConn2
  Line_7-8/RConn3 -- Bus_8 230 KV/RConn3
  "Bus_7 230 KV "/RConn3 -- Line_5-7/RConn3 -- Line_7-8/LConn3
  Load Flow Bus4/LConn1 -- "Bus_7 230 KV "/RConn1 -- Line_5-7/RConn1 -- Line_7-8/LConn1
  Generator BUS3x1/RConn1 -- Bus_3 13.8 KV/RConn1
  Line_5-7/RConn2 -- "Bus_7 230 KV "/RConn2 -- Line_7-8/LConn2
  Line_4-6/RConn1 -- 90 MW 30 MVAR/LConn1 -- Bus_6 230 KV/RConn1
  Line_4-5/RConn2 -- 125 MW 50 MVAR/LConn2 -- Bus_5 230 KV/RConn2
  Load Flow Bus/LConn1 -- Bus_1 16.5 KV/LConn1 -- "16.5 KV/230 KV 5.76 %Z     "/LConn1
  125 MW 50 MVAR/LConn1 -- Bus_5 230 KV/RConn1 -- Line_4-5/RConn1
  Line_4-5/RConn3 -- 125 MW 50 MVAR/LConn3 -- Bus_5 230 KV/RConn3
  Bus_8 230 KV/LConn2 -- 100 MW 35 MVAR/LConn2 -- Line_8-9/LConn2
  Bus_1 16.5 KV/LConn3 -- "16.5 KV/230 KV 5.76 %Z     "/LConn3
  Bus_1 16.5 KV/LConn2 -- "16.5 KV/230 KV 5.76 %Z     "/LConn2
  Bus_9 230 KV/RConn2 -- 13.8 KV/230 KV 5.86 %Z/RConn2
  Line_5-7/LConn2 -- Bus_5 230 KV/LConn2
  Bus_2 18 KV/RConn3 -- 18KV/230KV 6.25 %Z/LConn3
  Line_6-9/LConn2 -- Bus_6 230 KV/LConn2
  Line_4-6/LConn3 -- Line_4-5/LConn3 -- Bus_4 230 KV/RConn3 -- C/RConn1
  Generator BUS1x1/RConn1 -- Bus_1 16.5 KV/RConn1

== system WSCC_9bus_distributed/Interface_ss1_ss2/Subsystem1 ==
  sampler : Inport
  in2 : Inport  Port=2
  en2 : Inport  Port=3
  Demux1 : Demux  Outputs=[ -1 1 ]
  Manual Switch : ManualSwitch
  Mux : Mux  Inputs=2
  Network : CoSiF/Emulation/Network  Td=Td  Tdv=Tdv  Ts=Ts
      settings: SourceProductName=ACS Co-simulation Interfaces
  Switch1 : Switch  Criteria=u2 ~= 0  Threshold=0.5
  init right : CoSiF/Emulation/Interface/init left  k=1  mag=abs(init_right)*sqrt(2)/sqrt(3)  phase=rad2deg(phase(init_right))
      settings: SourceProductName=ACS Co-simulation Interfaces
  ou2 : Outport
  wires:
  en2/1 -> Mux/2
  sampler/1 -> Network/1
  Manual Switch/1 -> ou2/1
  in2/1 -> Mux/1, Manual Switch/1
  Demux1/2 -> Switch1/2  "en"
  Mux/1 -> Network/2
  Demux1/1 -> Switch1/1
  init right/1 -> Switch1/3
  Network/1 -> Demux1/1
  Switch1/1 -> Manual Switch/2

== system WSCC_9bus_distributed/Interface_ss1_ss2/Subsystem2 ==
  in1 : Inport
  en1 : Inport  Port=2
  In3 : Inport  Port=3
  Demux : Demux  Outputs=[ -1 1 ]
  Manual Switch1 : ManualSwitch
  Mux1 : Mux  Inputs=2
  Network1 : CoSiF/Emulation/Network  Td=Td  Tdv=Tdv  Ts=Ts
      settings: SourceProductName=ACS Co-simulation Interfaces
  Switch : Switch  Criteria=u2 ~= 0  Threshold=0.5
  init left : Subsystem  mask{k=1, mag=0, phase=0}
      mask prompts: mag "Magnitude"; phase "Phase (deg)"
      mask init:
      | if k > 1
      |    za = [ 0 0 mag phase+0   zeros(1,2*(k-1)) ];
      |    zb = [ 0 0 mag phase-120 zeros(1,2*(k-1)) ];
      |    zc = [ 0 0 mag phase+120 zeros(1,2*(k-1)) ];
      | elseif k == 0
      |    za = [ 0 0 ];
      |    zb = [ 0 0 ];
      | else    
      |    za = [ 0 0 mag phase+0 ];
      |    zb = [ 0 0 mag phase-120 ];
      |    zc = [ 0 0 mag phase+120 ];
      | end
      | 
      | set_param([gcb '/A'], 'Value', mat2str(za));
      | set_param([gcb '/B'], 'Value', mat2str(zb));
      | set_param([gcb '/C'], 'Value', mat2str(zc));
  ou1 : Outport
  wires:
  en1/1 -> Mux1/2
  Switch/1 -> Manual Switch1/2
  Mux1/1 -> Network1/2
  In3/1 -> Network1/1
  init left/1(init) -> Switch/3
  Network1/1 -> Demux/1
  Manual Switch1/1 -> ou1/1
  Demux/2 -> Switch/2  "en"
  Demux/1 -> Switch/1
  in1/1 -> Manual Switch1/1, Mux1/1

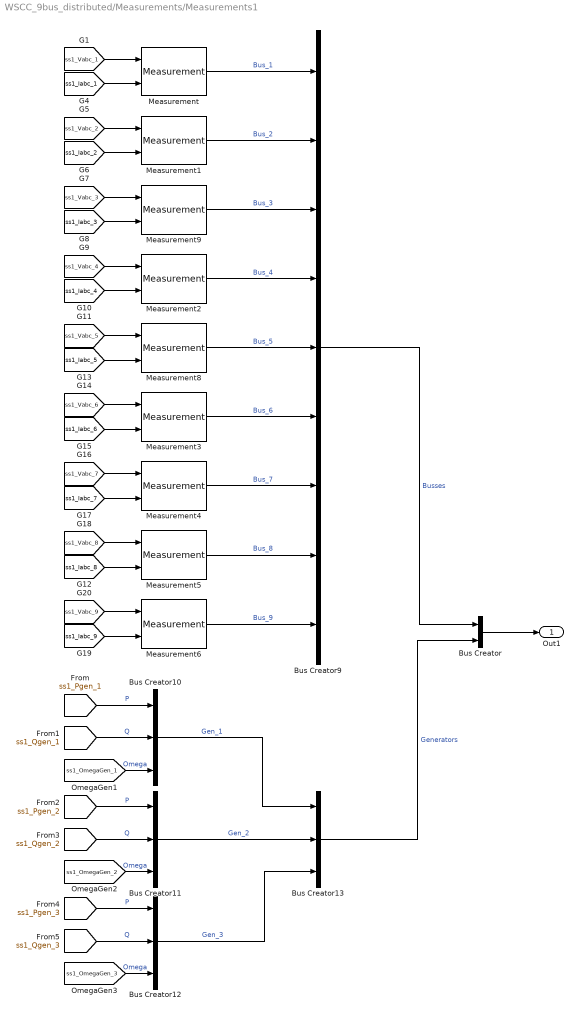
== system WSCC_9bus_distributed/Measurements/Measurements1 ==
  Bus Creator : BusCreator  Inputs=2
  Bus Creator{10..13} (4 alike) : BusCreator  Inputs=3
  Bus Creator9 : BusCreator  Inputs=9
  Measurement : library/Measurement  Vnom=16500
  Measurement1 : library/Measurement  Vnom=18000
  Measurement{2..6,8} (6 alike) : library/Measurement  Vnom=230000
  Measurement9 : library/Measurement  Vnom=13800
  Out1 : Outport
  wires:
  [ss1_Pgen_2] -> Bus Creator11/1  "P"
  [ss1_Qgen_3] -> Bus Creator12/2  "Q"
  [ss1_Qgen_2] -> Bus Creator11/2  "Q"
  [ss1_Qgen_1] -> Bus Creator10/2  "Q"
  [ss1_Pgen_1] -> Bus Creator10/1  "P"
  [ss1_OmegaGen_1] -> Bus Creator10/3  "Omega"
  [ss1_OmegaGen_2] -> Bus Creator11/3  "Omega"
  [ss1_Pgen_3] -> Bus Creator12/1  "P"
  [ss1_OmegaGen_3] -> Bus Creator12/3  "Omega"
  Bus Creator9/1 -> Bus Creator/1  "Busses"
  Bus Creator13/1 -> Bus Creator/2  "Generators"
  Bus Creator10/1 -> Bus Creator13/1  "Gen_1"
  Bus Creator11/1 -> Bus Creator13/2  "Gen_2"
  Bus Creator12/1 -> Bus Creator13/3  "Gen_3"
  Bus Creator/1 -> Out1/1
  [ss1_Vabc_1] -> Measurement/1
  [ss1_Iabc_1] -> Measurement/2
  Measurement/1 -> Bus Creator9/1  "Bus_1"
  [ss1_Iabc_2] -> Measurement1/2
  [ss1_Vabc_2] -> Measurement1/1
  [ss1_Vabc_3] -> Measurement9/1
  [ss1_Iabc_3] -> Measurement9/2
  [ss1_Vabc_4] -> Measurement2/1
  [ss1_Iabc_4] -> Measurement2/2
  [ss1_Iabc_5] -> Measurement8/2
  [ss1_Vabc_5] -> Measurement8/1
  [ss1_Vabc_6] -> Measurement3/1
  [ss1_Iabc_6] -> Measurement3/2
  [ss1_Iabc_9] -> Measurement6/2
  [ss1_Vabc_7] -> Measurement4/1
  [ss1_Iabc_7] -> Measurement4/2
  [ss1_Vabc_8] -> Measurement5/1
  [ss1_Iabc_8] -> Measurement5/2
  [ss1_Vabc_9] -> Measurement6/1
  Measurement6/1 -> Bus Creator9/9  "Bus_9"
  Measurement1/1 -> Bus Creator9/2  "Bus_2"
  Measurement9/1 -> Bus Creator9/3  "Bus_3"
  Measurement2/1 -> Bus Creator9/4  "Bus_4"
  Measurement8/1 -> Bus Creator9/5  "Bus_5"
  Measurement3/1 -> Bus Creator9/6  "Bus_6"
  Measurement4/1 -> Bus Creator9/7  "Bus_7"
  Measurement5/1 -> Bus Creator9/8  "Bus_8"

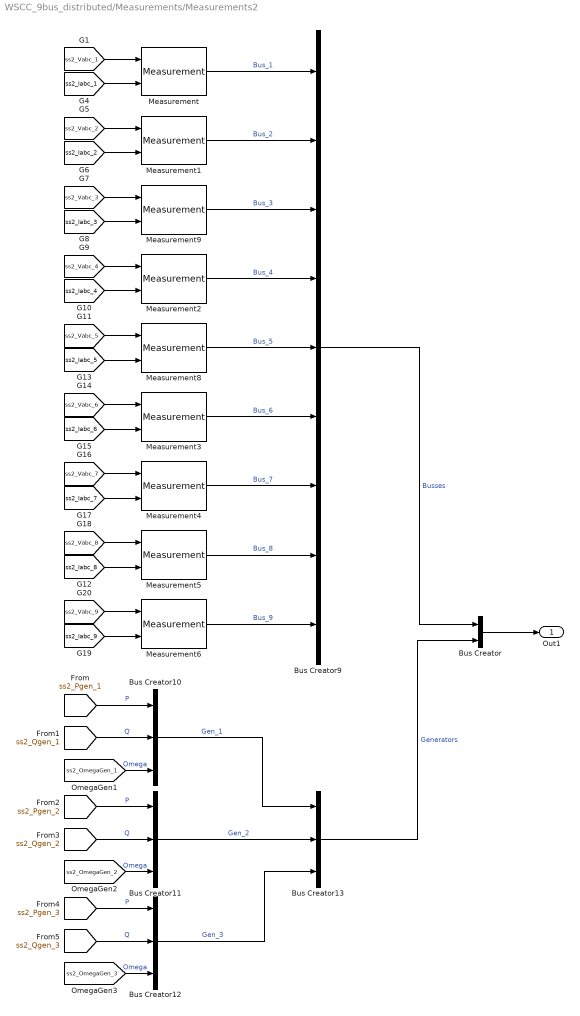
== system WSCC_9bus_distributed/Measurements/Measurements2 ==
  Bus Creator : BusCreator  Inputs=2
  Bus Creator{10..13} (4 alike) : BusCreator  Inputs=3
  Bus Creator9 : BusCreator  Inputs=9
  Measurement : library/Measurement  Vnom=16500
  Measurement1 : library/Measurement  Vnom=18000
  Measurement{2..6,8} (6 alike) : library/Measurement  Vnom=230000
  Measurement9 : library/Measurement  Vnom=13800
  Out1 : Outport
  wires:
  Measurement5/1 -> Bus Creator9/8  "Bus_8"
  Measurement4/1 -> Bus Creator9/7  "Bus_7"
  Measurement3/1 -> Bus Creator9/6  "Bus_6"
  Measurement8/1 -> Bus Creator9/5  "Bus_5"
  Measurement2/1 -> Bus Creator9/4  "Bus_4"
  Measurement9/1 -> Bus Creator9/3  "Bus_3"
  Measurement1/1 -> Bus Creator9/2  "Bus_2"
  Measurement6/1 -> Bus Creator9/9  "Bus_9"
  [ss2_Vabc_9] -> Measurement6/1
  [ss2_Iabc_8] -> Measurement5/2
  [ss2_Vabc_8] -> Measurement5/1
  [ss2_Iabc_7] -> Measurement4/2
  [ss2_Vabc_7] -> Measurement4/1
  [ss2_Iabc_9] -> Measurement6/2
  [ss2_Iabc_6] -> Measurement3/2
  [ss2_Vabc_6] -> Measurement3/1
  [ss2_Vabc_5] -> Measurement8/1
  [ss2_Iabc_5] -> Measurement8/2
  [ss2_Iabc_4] -> Measurement2/2
  [ss2_Vabc_4] -> Measurement2/1
  [ss2_Iabc_3] -> Measurement9/2
  [ss2_Vabc_3] -> Measurement9/1
  [ss2_Vabc_2] -> Measurement1/1
  [ss2_Iabc_2] -> Measurement1/2
  Measurement/1 -> Bus Creator9/1  "Bus_1"
  [ss2_Iabc_1] -> Measurement/2
  [ss2_Vabc_1] -> Measurement/1
  Bus Creator/1 -> Out1/1
  Bus Creator12/1 -> Bus Creator13/3  "Gen_3"
  Bus Creator11/1 -> Bus Creator13/2  "Gen_2"
  Bus Creator10/1 -> Bus Creator13/1  "Gen_1"
  Bus Creator13/1 -> Bus Creator/2  "Generators"
  Bus Creator9/1 -> Bus Creator/1  "Busses"
  [ss2_OmegaGen_3] -> Bus Creator12/3  "Omega"
  [ss2_Pgen_3] -> Bus Creator12/1  "P"
  [ss2_OmegaGen_2] -> Bus Creator11/3  "Omega"
  [ss2_OmegaGen_1] -> Bus Creator10/3  "Omega"
  [ss2_Pgen_1] -> Bus Creator10/1  "P"
  [ss2_Qgen_1] -> Bus Creator10/2  "Q"
  [ss2_Qgen_2] -> Bus Creator11/2  "Q"
  [ss2_Qgen_3] -> Bus Creator12/2  "Q"
  [ss2_Pgen_2] -> Bus Creator11/1  "P"

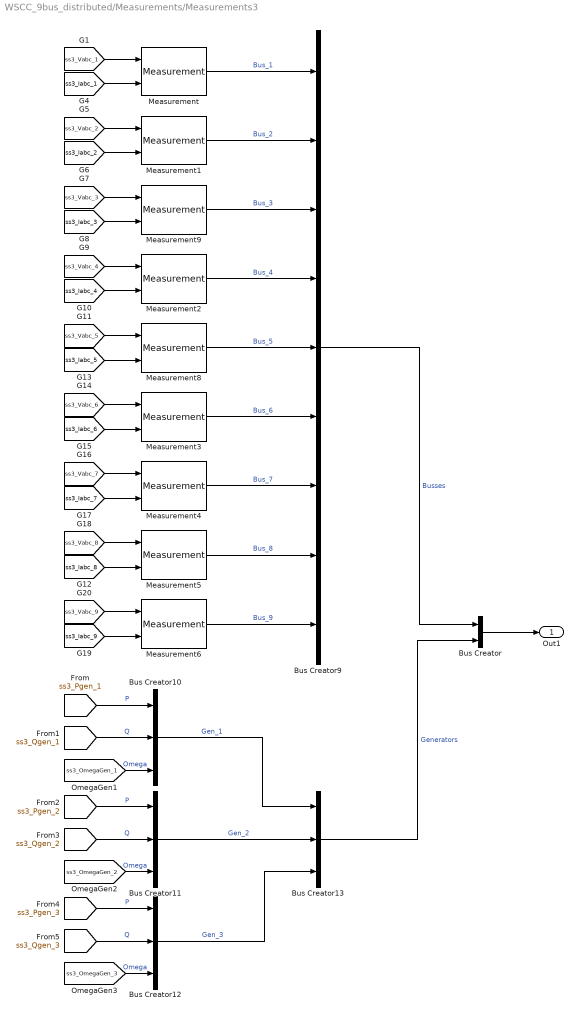
== system WSCC_9bus_distributed/Measurements/Measurements3 ==
  Bus Creator : BusCreator  Inputs=2
  Bus Creator{10..13} (4 alike) : BusCreator  Inputs=3
  Bus Creator9 : BusCreator  Inputs=9
  Measurement : library/Measurement  Vnom=16500
  Measurement1 : library/Measurement  Vnom=18000
  Measurement{2..6,8} (6 alike) : library/Measurement  Vnom=230000
  Measurement9 : library/Measurement  Vnom=13800
  Out1 : Outport
  wires:
  [ss3_Pgen_2] -> Bus Creator11/1  "P"
  [ss3_Qgen_3] -> Bus Creator12/2  "Q"
  [ss3_Qgen_2] -> Bus Creator11/2  "Q"
  [ss3_Qgen_1] -> Bus Creator10/2  "Q"
  [ss3_Pgen_1] -> Bus Creator10/1  "P"
  [ss3_OmegaGen_1] -> Bus Creator10/3  "Omega"
  [ss3_OmegaGen_2] -> Bus Creator11/3  "Omega"
  [ss3_Pgen_3] -> Bus Creator12/1  "P"
  [ss3_OmegaGen_3] -> Bus Creator12/3  "Omega"
  Bus Creator9/1 -> Bus Creator/1  "Busses"
  Bus Creator13/1 -> Bus Creator/2  "Generators"
  Bus Creator10/1 -> Bus Creator13/1  "Gen_1"
  Bus Creator11/1 -> Bus Creator13/2  "Gen_2"
  Bus Creator12/1 -> Bus Creator13/3  "Gen_3"
  Bus Creator/1 -> Out1/1
  [ss3_Vabc_1] -> Measurement/1
  [ss3_Iabc_1] -> Measurement/2
  Measurement/1 -> Bus Creator9/1  "Bus_1"
  [ss3_Iabc_2] -> Measurement1/2
  [ss3_Vabc_2] -> Measurement1/1
  [ss3_Vabc_3] -> Measurement9/1
  [ss3_Iabc_3] -> Measurement9/2
  [ss3_Vabc_4] -> Measurement2/1
  [ss3_Iabc_4] -> Measurement2/2
  [ss3_Iabc_5] -> Measurement8/2
  [ss3_Vabc_5] -> Measurement8/1
  [ss3_Vabc_6] -> Measurement3/1
  [ss3_Iabc_6] -> Measurement3/2
  [ss3_Iabc_9] -> Measurement6/2
  [ss3_Vabc_7] -> Measurement4/1
  [ss3_Iabc_7] -> Measurement4/2
  [ss3_Vabc_8] -> Measurement5/1
  [ss3_Iabc_8] -> Measurement5/2
  [ss3_Vabc_9] -> Measurement6/1
  Measurement6/1 -> Bus Creator9/9  "Bus_9"
  Measurement1/1 -> Bus Creator9/2  "Bus_2"
  Measurement9/1 -> Bus Creator9/3  "Bus_3"
  Measurement2/1 -> Bus Creator9/4  "Bus_4"
  Measurement8/1 -> Bus Creator9/5  "Bus_5"
  Measurement3/1 -> Bus Creator9/6  "Bus_6"
  Measurement4/1 -> Bus Creator9/7  "Bus_7"
  Measurement5/1 -> Bus Creator9/8  "Bus_8"

== system WSCC_9bus_distributed/Measurements/Scopes ==
  In1 : Inport
  Bus Selector12 : BusSelector  OutputSignals=SS1.Generators.Gen_2.Omega,SS1.Generators.Gen_1.Omega,SS1.Generators.Gen_3.Omega,SS2.Generators.Gen_2.Omega,SS2.Generators.Gen_1.Omega,SS2.Generators.Gen_3.Omega
  Bus Selector9 : BusSelector  OutputSignals=SS1,SS2
  Generators : Scope  NumInputPorts=6
  Scopes SS1 : Subsystem
  Scopes SS2 : Subsystem
  wires:
  Bus Selector12/3 -> Generators/3  "<Omega>"
  Bus Selector12/5 -> Generators/5  "<Omega>"
  In1/1 -> Bus Selector9/1, Bus Selector12/1
  Bus Selector12/1 -> Generators/1  "<Omega>"
  Bus Selector12/6 -> Generators/6  "<Omega>"
  Bus Selector12/2 -> Generators/2  "<Omega>"
  Bus Selector12/4 -> Generators/4  "<Omega>"
  Bus Selector9/1 -> Scopes SS1/1(In1)  "<SS1>"
  Bus Selector9/2 -> Scopes SS2/1(In1)  "<SS2>"

== system WSCC_9bus_distributed/Measurements/Scopes1 ==
  In1 : Inport
  Bus Selector1 : BusSelector  OutputSignals=Busses.Bus_2.Vrms  OutputAsBus=on
  Bus Selector10 : BusSelector  OutputSignals=Busses.Bus_1.Vrms  OutputAsBus=on
  Bus Selector12 : BusSelector  OutputSignals=SS1.Generators.Gen_2.Omega,SS1.Generators.Gen_1.Omega,SS1.Generators.Gen_3.Omega,SS2.Generators.Gen_2.Omega,SS2.Generators.Gen_1.Omega,SS2.Generators.Gen_3.Omega,SS3.Generators.Gen_1.Omega,SS3.Generators.Gen_2.Omega,SS3.Generators.Gen_3.Omega
  Bus Selector2 : BusSelector  OutputSignals=Busses.Bus_3.Vrms  OutputAsBus=on
  Bus Selector3 : BusSelector  OutputSignals=Busses.Bus_4.Vrms  OutputAsBus=on
  Bus Selector4 : BusSelector  OutputSignals=Busses.Bus_5.Vrms  OutputAsBus=on
  Bus Selector5 : BusSelector  OutputSignals=Busses.Bus_6.Vrms  OutputAsBus=on
  Bus Selector6 : BusSelector  OutputSignals=Busses.Bus_7.Vrms  OutputAsBus=on
  Bus Selector7 : BusSelector  OutputSignals=Busses.Bus_8.Vrms  OutputAsBus=on
  Bus Selector8 : BusSelector  OutputSignals=Busses.Bus_9.Vrms  OutputAsBus=on
  Bus Selector9 : BusSelector  OutputSignals=SS1
  Generators : Scope  NumInputPorts=9
  Voltages : Scope  NumInputPorts=9
  wires:
  Bus Selector12/7 -> Generators/7  "<Omega>"
  Bus Selector12/8 -> Generators/8  "<Omega>"
  Bus Selector12/9 -> Generators/9  "<Omega>"
  Bus Selector12/4 -> Generators/4  "<Omega>"
  Bus Selector12/2 -> Generators/2  "<Omega>"
  Bus Selector3/1 -> Voltages/4  "Bus_4"
  Bus Selector12/6 -> Generators/6  "<Omega>"
  Bus Selector12/1 -> Generators/1  "<Omega>"
  In1/1 -> Bus Selector12/1, Bus Selector9/1
  Bus Selector2/1 -> Voltages/3  "Bus_3"
  Bus Selector12/5 -> Generators/5  "<Omega>"
  Bus Selector6/1 -> Voltages/7  "Bus_7"
  Bus Selector9/1 -> Bus Selector10/1, Bus Selector1/1, Bus Selector2/1, Bus Selector3/1, Bus Selector7/1, Bus Selector8/1, Bus Selector6/1, Bus Selector5/1, Bus Selector4/1  "<SS1>"
  Bus Selector12/3 -> Generators/3  "<Omega>"
  Bus Selector1/1 -> Voltages/2  "Bus_2"
  Bus Selector8/1 -> Voltages/9  "Bus_9"
  Bus Selector5/1 -> Voltages/6  "Bus_6"
  Bus Selector10/1 -> Voltages/1  "Bus_1"
  Bus Selector4/1 -> Voltages/5  "Bus_5"
  Bus Selector7/1 -> Voltages/8  "Bus_8"
